simulink model "NHR9200Model4960_2020b_prog"  (R2020b)
settings: Solver=ode23tb  StartTime=0.0  StopTime=tFinal  FixedStep=Ts  MaxStep=0.2  RelTol=1e-3
values from neighbouring files (symbols this model uses):
  Imax_snk = 40    [nhr9200_runProg.m]
  Imax_snk_sfty = 80    [nhr9200_runProg.m]
  Imax_src = 10    [nhr9200_runProg.m]
  Imax_src_sfty = 25    [nhr9200_runProg.m]
  nhrLoad = 15    [nhr9200_runProg.m]
  op_state = 2    [nhr9200_runProg.m]
  Pmax_snk = 12    [nhr9200_runProg.m]
  Pmax_snk_sfty = 800    [nhr9200_runProg.m]
  Pmax_src = 8    [nhr9200_runProg.m]
  Pmax_src_sfty = 5000    [nhr9200_runProg.m]
  R_src = 0.001    [nhr9200_runProg.m]
  slew_i = 10    [nhr9200_runProg.m]
  slew_p = 300    [nhr9200_runProg.m]
  slew_r = 400    [nhr9200_runProg.m]
  slew_v = 200    [nhr9200_runProg.m]
  t_Imax_snk_sfty = 2    [nhr9200_runProg.m]
  t_Imax_src_sfty = 0.5    [nhr9200_runProg.m]
  t_Pmax_snk_sfty = 2    [nhr9200_runProg.m]
  t_Pmax_src_sfty = 2    [nhr9200_runProg.m]
  t_Vmax_gb = 2    [nhr9200_runProg.m]
  t_Vmin_gb = 2    [nhr9200_runProg.m]
  turn_on = 1    [nhr9200_runProg.m]
  v_bat = 0    [nhr9200_runProg.m]
  Vmax_gb = 800    [nhr9200_runProg.m]
  Vmax_src = 480    [nhr9200_runProg.m]
  Vmin_gb = -50    [nhr9200_runProg.m]
  Vmin_snk = 20    [nhr9200_runProg.m]
libraries: simulink x31, fl_lib x15, nesl_utility x14, simulink_extras x6, powerlib_meascontrol x6, ee_lib x2
(part 1 of 2)
settings Model: Creator=opal  LastModifiedBy=mne4
settings DataIOCC: ReturnWorkspaceOutputs=off
settings DebuggingCC: ParameterPrecisionLossMsg=none  UnconnectedInputMsg=none  UnconnectedOutputMsg=none  UnconnectedLineMsg=none  ArithmeticOperatorsInVariantConditions=warning
settings SFSimCC: SimUseLocalCustomCode=off  CustomCodeUndefinedFunction=UseInterfaceOnly
settings RTWCC: RTWUseLocalCustomCode=off
settings CodeAppCC: StateflowObjectComments=on
settings SimscapeCC: SimscapeNormalizeSystem=off

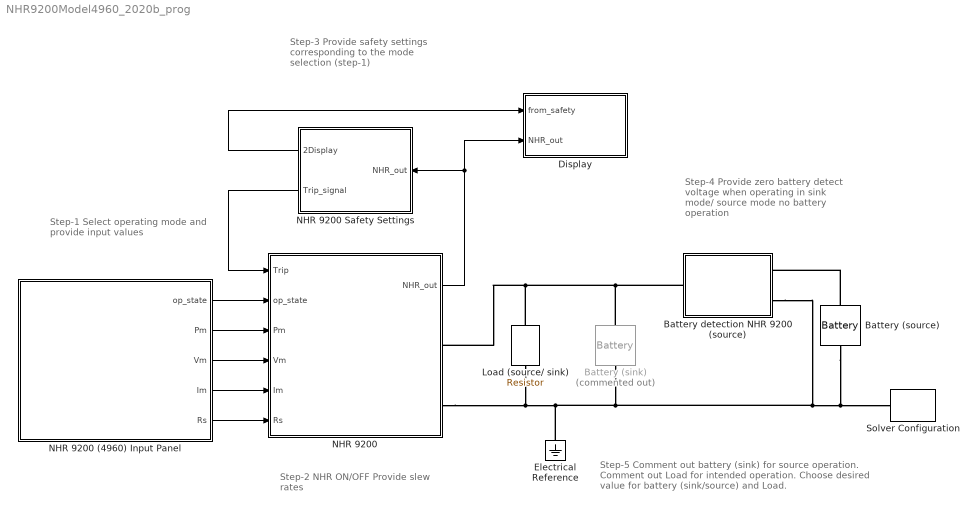
== system NHR9200Model4960_2020b_prog ==
  note: Step-1
      | Select operating mode and provide input values
  note: Step-2
      | NHR ON/OFF
      | Provide slew rates
  note: Step-3
      | Provide safety settings corresponding to the mode selection (step-1)
  note: Step-4
      | Provide zero battery detect voltage when operating in sink mode/ source mode no battery operation
  note: Step-5
      | Comment out battery (sink) for source operation.
      | Comment out Load for intended operation.
      | Choose desired value for battery (sink/source) and Load.
  Battery (sink) : ee_lib/Sources/Battery  Commented=on  Vnom=v_nom_bat_snk V  prm_dir=1  R1_dis=2 Ohm  R1_ch=2 Ohm  R1=r_bat_snk Ohm  prm_AH=1  AH=50 hr*A  V1=11.5 V  AH1=25 hr*A  prm_R2=1  R2=2000 Ohm  prm_dyn=1  Rp1=0.005 Ohm  tau1=30 s  Rp2=0.005 Ohm  tau2=30 s  Rp3=0.005 Ohm  tau3=30 s  Rp4=0.005 Ohm  tau4=30 s  Rp5=0.005 Ohm  tau5=30 s  prm_fade=1  N_fade=100  AH_fade=45 hr*A  R1_fade=2.02 Ohm  R1_ch_fade=2.02 Ohm  V1_fade=10.35 V  i_specify=off  i_priority=None  i=0 A  i_nominal_specify=off  i_nominal_unit=A  i_nominal_value=1  v_specify=off  v_priority=None  v=0 V  v_nominal_specify=off  v_nominal_unit=V  v_nominal_value=1  charge_specify=off  charge_priority=High  charge=50 hr*A  charge_nominal_specify=off  charge_nominal_unit=hr*A  charge_nominal_value=1  num_cycles_specify=off  num_cycles_priority=High  num_cycles=0  num_cycles_nominal_specify=off  num_cycles_nominal_unit=1  num_cycles_nominal_value=1  thermal_mass=30000 J/K  Tmeas=298.15 K  Vnom_T2=12 V  R1_T2=2.2 Ohm  R1_T2_dis=2.2 Ohm  R1_T2_ch=2.2 Ohm  V1_T2=11.4 V  R2_T2=2200 Ohm  Rp1_T2=0.005 Ohm  tau1_T2=30 s  Rp2_T2=0.005 Ohm  tau2_T2=30 s  Rp3_T2=0.005 Ohm  tau3_T2=30 s  Rp4_T2=0.005 Ohm  tau4_T2=30 s  Rp5_T2=0.005 Ohm  tau5_T2=30 s  Tmeas2=273.15 K  temperature_specify=off  temperature_priority=High  temperature=298.15 K  temperature_nominal_specify=off  temperature_nominal_unit=K  temperature_nominal_value=1
  Battery (source) : ee_lib/Sources/Battery  Vnom=v_nom_bat_src V  prm_dir=1  R1_dis=2 Ohm  R1_ch=2 Ohm  R1=r_bat_src Ohm  prm_AH=1  AH=50 hr*A  V1=11.5 V  AH1=25 hr*A  prm_R2=1  R2=2000 Ohm  prm_dyn=1  Rp1=0.005 Ohm  tau1=30 s  Rp2=0.005 Ohm  tau2=30 s  Rp3=0.005 Ohm  tau3=30 s  Rp4=0.005 Ohm  tau4=30 s  Rp5=0.005 Ohm  tau5=30 s  prm_fade=1  N_fade=100  AH_fade=45 hr*A  R1_fade=2.02 Ohm  R1_ch_fade=2.02 Ohm  V1_fade=10.35 V  i_specify=off  i_priority=None  i=0 A  i_nominal_specify=off  i_nominal_unit=A  i_nominal_value=1  v_specify=off  v_priority=None  v=0 V  v_nominal_specify=off  v_nominal_unit=V  v_nominal_value=1  charge_specify=off  charge_priority=High  charge=50 hr*A  charge_nominal_specify=off  charge_nominal_unit=hr*A  charge_nominal_value=1  num_cycles_specify=off  num_cycles_priority=High  num_cycles=0  num_cycles_nominal_specify=off  num_cycles_nominal_unit=1  num_cycles_nominal_value=1  thermal_mass=30000 J/K  Tmeas=298.15 K  Vnom_T2=12 V  R1_T2=2.2 Ohm  R1_T2_dis=2.2 Ohm  R1_T2_ch=2.2 Ohm  V1_T2=11.4 V  R2_T2=2200 Ohm  Rp1_T2=0.005 Ohm  tau1_T2=30 s  Rp2_T2=0.005 Ohm  tau2_T2=30 s  Rp3_T2=0.005 Ohm  tau3_T2=30 s  Rp4_T2=0.005 Ohm  tau4_T2=30 s  Rp5_T2=0.005 Ohm  tau5_T2=30 s  Tmeas2=273.15 K  temperature_specify=off  temperature_priority=High  temperature=298.15 K  temperature_nominal_specify=off  temperature_nominal_unit=K  temperature_nominal_value=1
  Battery detection NHR 9200 (source) : Subsystem  mask{Vdetect=v_bat}
      mask prompts: Vdetect "Battery detect voltage: (0: battery detection disabled)"
  Display : Subsystem
  Electrical Reference : fl_lib/Electrical/Electrical Elements/Electrical Reference
  Load (source/ sink) : fl_lib/Electrical/Electrical Elements/Resistor  R=nhrLoad Ohm  i_specify=off  i_priority=None  i=0 A  i_nominal_specify=off  i_nominal_unit=A  i_nominal_value=1  v_specify=off  v_priority=None  v=0 V  v_nominal_specify=off  v_nominal_unit=V  v_nominal_value=1
  NHR 9200 : Subsystem  mask{p_switch=turn_on, Vslew=slew_v, Islew=slew_i, Rslew=slew_r, Pslew=slew_p, Vbset=v_bat}
      mask prompts: p_switch "Enter 1 to turn ON, 0 to turn OFF NHR 9200"
      mask DialogControl DescTextVar Prompt: NHR 9200
      mask DialogControl Container5 Prompt: Slew Rates
      mask DialogControl control2 Prompt: Voltage slew rate [0.165V/s-600V/ms]:
      mask DialogControl Control3 Prompt: Current slew rate [0.011 A/s-40A/ms]:
      mask DialogControl Control4 Prompt: Resistance slew rate [0.14 ohms/s-500 ohms/ms]:
      mask DialogControl Control5 Prompt: Power slew rate [2W/s-8kW/s]:
      mask DialogControl Container6 Prompt: Set Battery Detect Voltage
      mask DialogControl Control7 Prompt: Battery detect voltage: (0: battery detection disabled)
      mask Display: image('NHR9200.png');
  NHR 9200 (4960) Input Panel : Subsystem  mask{op_state=op_state, Vmch=Vmax_src, Imch=Imax_src, Pmch=Pmax_src, Rsch=R_src, Vmdch=Vmin_snk, Imdch=Imax_snk, Pmdch=Pmax_snk}
      mask DialogControl Control2 Prompt: Select operating state (1: standby, 2: Charge, 3: Discharge, 4: Battery)
      mask DialogControl Container7 Prompt: Limiting mode (CV, CC, CP, CR)
      mask DialogControl Container9 Prompt: Set '0' to disable a mode
      mask DialogControl Container4 Prompt: Charging mode input parameters
      mask DialogControl Control3 Prompt: Max Voltage [0~600V]:
      mask DialogControl Control4 Prompt: Max Current [0~(+40)A]:
      mask DialogControl Control5 Prompt: Max Power [0~8kW]:
      mask DialogControl Control6 Prompt: Resistance [0~500 ohms]:
      mask DialogControl Container4_copy Prompt: Discharging mode input parameters
      mask DialogControl Control3_copy Prompt: Min Voltage [10~600V]:
      mask DialogControl Control4_copy Prompt: Max Current [0~(-40)A], enter absolute value:
      mask DialogControl Control5_copy Prompt: Max Power [0~12kW]:
      mask Display: image('NHR9200Model4960HMI.png');
  NHR 9200 Safety Settings : Subsystem  mask{Vmin=Vmin_gb, Tvmin=t_Vmin_gb, Vmax=Vmax_gb, Tvmax=t_Vmax_gb, Imaxdch=Imax_snk_sfty, Timaxdch=t_Imax_snk_sfty, Pmaxdch=Pmax_snk_sfty, Tpmaxdch=t_Pmax_snk_sfty, Imaxch=Imax_src_sfty, Timaxch=t_Imax_src_sfty, Pmaxch=Pmax_src_sfty, Tpmaxch=t_Pmax_src_sfty}
      mask prompts: Vmin "Min Voltage (V):"; Tvmin "Min Voltage time (S):"; Vmax "Max Voltage (V):"; Tvmax "Max Voltage time (S):"; Imaxdch "Max Current (A):"; Timaxdch "Max Current Time (S):"; Pmaxdch "Max Power (W):"; Tpmaxdch "Max Power Time (S):"; Imaxch "Max Current (A):"; Timaxch "Max Current Time (S):"; Pmaxch "Max Power (W):"; Tpmaxch "Max Power Time (S):"
      mask DialogControl DescTextVar Prompt: NHR 9410 Safety Settings
      mask DialogControl Container27 Prompt: Provide safety trip parameters
      mask DialogControl Container123 Prompt: Global safety limits (all modes)
      mask DialogControl Container124 Prompt: Discharge safety limits (sink mode- discharge and battery)
      mask DialogControl Container125 Prompt: Charge safety limits (source mode- charge and battery)
  Solver Configuration : nesl_utility/Solver Configuration  PhysicalDomain=network_engine_domain  SubClassName=solver  LeftPortType=input  RightPortType=generic  Tones=[]  Harmonics=[]  SimulateNoise=off  Profile=off  UseLocalSampling=off  EnableSwitchedLinearOptims=on  FrequencyDomain=off  UseCCode=off  RelTol=0.001  AbsTol=1e-06  MinStep=1e-09  ToWorkspace=off  RevertToSquareIcSolve=off  NumHomotopyIterations=100  PhasorMode=off  PhasorModeNumHarmonics=1  DoDC=off  ResidualTolerance=1e-09  UseLocalSolver=on  LocalSolverChoice=NE_TRAPEZOIDAL_ADVANCER  LocalSolverSampleTime=Ts  DoFixedCost=off  MaxNonlinIter=3  MaxModeIter=2  ComputeImpulses=off  ImpulseIterations=2  LinearAlgebra=Sparse  EquationFormulation=NE_TIME_EF  DelaysMemoryBudget=1024  AutomaticFiltering=off  FilteringTimeConstant=0.001  PartitionStorageMethod=AS_NEEDED  PartitionMemoryBudget=1024  PartitionMethod=FAST
  wires:
  NHR 9200/1(NHR_out) -> Display/2(NHR_out), NHR 9200 Safety Settings/1(NHR_out)
  NHR 9200 Safety Settings/2(Trip_signal) -> NHR 9200/1(Trip)
  NHR 9200 (4960) Input Panel/1(op_state) -> NHR 9200/2(op_state)
  NHR 9200 (4960) Input Panel/2(Pm) -> NHR 9200/3(Pm)
  NHR 9200 (4960) Input Panel/3(Vm) -> NHR 9200/4(Vm)
  NHR 9200 (4960) Input Panel/4(Im) -> NHR 9200/5(Im)
  NHR 9200 (4960) Input Panel/5(Rs) -> NHR 9200/6(Rs)
  NHR 9200 Safety Settings/1(2Display) -> Display/1(from_safety)
  connections:
  Electrical Reference/LConn1 -- NHR 9200/RConn2 -- Load (source/ sink)/RConn1 -- Battery detection NHR 9200 (source)/LConn2 -- Battery (source)/RConn1 -- Solver Configuration/RConn1 -- Battery (sink)/RConn1
  Load (source/ sink)/LConn1 -- Battery (sink)/LConn1 -- Battery detection NHR 9200 (source)/RConn1 -- NHR 9200/RConn1
  Battery (source)/LConn1 -- Battery detection NHR 9200 (source)/LConn1

== system NHR9200Model4960_2020b_prog/Battery detection NHR 9200 (source) ==
  Battery detection : Subsystem
  Switch : fl_lib/Electrical/Electrical Elements/Switch  R_closed=1e-6 Ohm  G_open=1e-50 1/Ohm  Threshold=0.5  i_specify=off  i_priority=None  i=0 A  i_nominal_specify=off  i_nominal_unit=A  i_nominal_value=1  v_specify=off  v_priority=None  v=0 V  v_nominal_specify=off  v_nominal_unit=V  v_nominal_value=1
  Voltage Sensor : fl_lib/Electrical/Electrical Sensors/Voltage Sensor
  +in : PMIOPort  Side=Right
  +out2battery : PMIOPort  Port=2  Side=Left
  - : PMIOPort  Port=3  Side=Left
  connections:
  Voltage Sensor/LConn1 -- +out2battery/RConn1 -- Switch/LConn1
  Battery detection/LConn1 -- Voltage Sensor/RConn1
  Switch/RConn2 -- +in/RConn1
  Battery detection/RConn1 -- Switch/RConn1
  Voltage Sensor/RConn2 -- -/RConn1

== system NHR9200Model4960_2020b_prog/Display ==
  note: Pmax_trip (charge)
  note: Imax_trip (charge)
  note: Pmax_trip (discharge)
  note: Imax_trip (discharge)
  note: Vmax_trip
  note: Vmin_trip
  note: Trip
  from_safety : Inport
  NHR_out : Inport  Port=2
  Demux : Demux
  Demux1 : Demux  Outputs=7
  Divide : Product  Commented=on  Inputs=*/
  Mux : Mux  Inputs=2
  NHR 9200 output waveforms [P,V,I] : Scope  NumInputPorts=3
  R : Scope  Commented=on
  Terminator : Terminator
  Trip Signals : Scope  NumInputPorts=7
  Vout/Vuut : Scope  NumInputPorts=2
  wires:
  Demux/1 -> NHR 9200 output waveforms [P,V,I]/1
  NHR_out/1 -> Demux/1
  from_safety/1 -> Demux1/1
  Demux1/1 -> Trip Signals/1
  Demux1/2 -> Trip Signals/2
  Demux1/3 -> Trip Signals/3
  Demux1/4 -> Trip Signals/4
  Demux1/5 -> Trip Signals/5
  Demux1/6 -> Trip Signals/6
  Demux1/7 -> Trip Signals/7
  Demux/4 -> Terminator/1
  Demux/2 -> Mux/1, Divide/1, NHR 9200 output waveforms [P,V,I]/2
  Divide/1 -> R/1
  Demux/3 -> Divide/2, NHR 9200 output waveforms [P,V,I]/3
  [Vuut_bat] -> Mux/2
  [Vdetect] -> Vout/Vuut/2
  Mux/1 -> Vout/Vuut/1

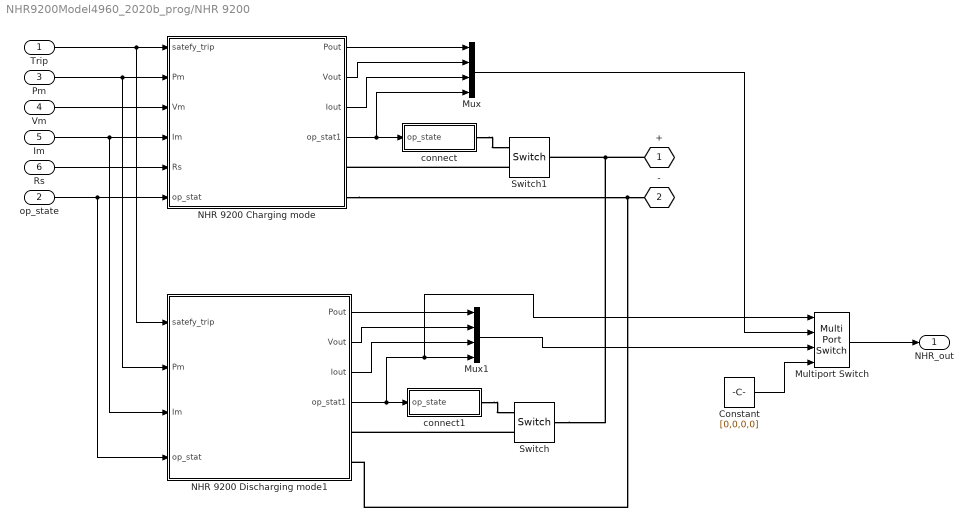
== system NHR9200Model4960_2020b_prog/NHR 9200 ==
  Trip : Inport
  op_state : Inport  Port=2
  Pm : Inport  Port=3
  Vm : Inport  Port=4
  Im : Inport  Port=5
  Rs : Inport  Port=6
  Constant : Constant  Value=[0,0,0,0]
  Multiport Switch : MultiPortSwitch  DataPortOrder=Specify indices  Inputs=2  DataPortIndices={2,3}  DataPortForDefault=Additional data port  DiagnosticForDefault=None
  Mux : Mux
  Mux1 : Mux
  NHR 9200 Charging mode : Subsystem
  NHR 9200 Discharging mode1 : Subsystem
  Switch : fl_lib/Electrical/Electrical Elements/Switch  R_closed=1e-6 Ohm  G_open=1e-50 1/Ohm  Threshold=0.5  i_specify=off  i_priority=None  i=0 A  i_nominal_specify=off  i_nominal_unit=A  i_nominal_value=1  v_specify=off  v_priority=None  v=0 V  v_nominal_specify=off  v_nominal_unit=V  v_nominal_value=1
  Switch1 : fl_lib/Electrical/Electrical Elements/Switch  R_closed=1e-6 Ohm  G_open=1e-50 1/Ohm  Threshold=0.5  i_specify=off  i_priority=None  i=0 A  i_nominal_specify=off  i_nominal_unit=A  i_nominal_value=1  v_specify=off  v_priority=None  v=0 V  v_nominal_specify=off  v_nominal_unit=V  v_nominal_value=1
  connect : Subsystem  mask{op_state=2}
      mask prompts: op_state "Intended operating state (integer number):"
      mask DialogControl Control3 Prompt: Select operating state (1: standby, 2: Charge, 3: Discharge, 4: Battery)
  connect1 : Subsystem  mask{op_state=3}
      mask prompts: op_state "Intended operating state (integer number):"
      mask DialogControl Control3 Prompt: Select operating state (1: standby, 2: Charge, 3: Discharge, 4: Battery)
  + : PMIOPort  Side=Right
  - : PMIOPort  Port=2  Side=Right
  NHR_out : Outport  VectorParamsAs1DForOutWhenUnconnected=off
  wires:
  Vm/1 -> NHR 9200 Charging mode/3(Vm)
  Im/1 -> NHR 9200 Discharging mode1/3(Im), NHR 9200 Charging mode/4(Im)
  Rs/1 -> NHR 9200 Charging mode/5(Rs)
  NHR 9200 Charging mode/1(Pout) -> Mux/1
  NHR 9200 Charging mode/2(Vout) -> Mux/2
  NHR 9200 Charging mode/3(Iout) -> Mux/3
  op_state/1 -> NHR 9200 Discharging mode1/4("op_stat "), NHR 9200 Charging mode/6("op_stat ")
  Trip/1 -> NHR 9200 Discharging mode1/1(satefy_trip), NHR 9200 Charging mode/1(satefy_trip)
  NHR 9200 Charging mode/4(op_stat1) -> Mux/4, connect/1(op_state)
  Pm/1 -> NHR 9200 Discharging mode1/2(Pm), NHR 9200 Charging mode/2(Pm)
  NHR 9200 Discharging mode1/4(op_stat1) -> Mux1/4, Multiport Switch/1, connect1/1(op_state)
  NHR 9200 Discharging mode1/3(Iout) -> Mux1/3
  NHR 9200 Discharging mode1/2(Vout) -> Mux1/2
  NHR 9200 Discharging mode1/1(Pout) -> Mux1/1
  Multiport Switch/1 -> NHR_out/1
  Mux1/1 -> Multiport Switch/3
  Mux/1 -> Multiport Switch/2
  Constant/1 -> Multiport Switch/4
  connections:
  NHR 9200 Discharging mode1/RConn2 -- NHR 9200 Charging mode/RConn2 -- -/RConn1
  +/RConn1 -- Switch/LConn1 -- Switch1/LConn1
  Switch1/RConn2 -- NHR 9200 Charging mode/RConn1
  connect/RConn1 -- Switch1/RConn1
  connect1/RConn1 -- Switch/RConn1
  Switch/RConn2 -- NHR 9200 Discharging mode1/RConn1

== system NHR9200Model4960_2020b_prog/NHR 9200 (4960) Input Panel ==
  Charging mode Input Params : Subsystem
  Compare To Constant1 : simulink/Logic and Bit Operations/Compare To Constant  relop===  const=3  OutDataTypeStr=boolean
  Compare To Constant4 : simulink/Logic and Bit Operations/Compare To Constant  relop===  const=2  OutDataTypeStr=boolean
  Constant : Constant  Value=op_state
  Constant1 : Constant  Value=[0,0,0,0]
  Demux : Demux
  Discharging mode Input Params : Subsystem
  Multiport Switch : MultiPortSwitch  DataPortOrder=Specify indices  Inputs=2  DataPortIndices={2,3}  DataPortForDefault=Additional data port  DiagnosticForDefault=None
  Mux : Mux
  Mux1 : Mux
  op_state : Outport  VectorParamsAs1DForOutWhenUnconnected=off
  Pm : Outport  Port=2  VectorParamsAs1DForOutWhenUnconnected=off
  Vm : Outport  Port=3  VectorParamsAs1DForOutWhenUnconnected=off
  Im : Outport  Port=4  VectorParamsAs1DForOutWhenUnconnected=off
  Rs : Outport  Port=5  VectorParamsAs1DForOutWhenUnconnected=off
  wires:
  Compare To Constant4/1 -> Charging mode Input Params/Enable
  Constant/1 -> Compare To Constant1/1, Multiport Switch/1, op_state/1, Compare To Constant4/1
  Demux/1 -> Vm/1
  Demux/2 -> Im/1
  Demux/3 -> Pm/1
  Demux/4 -> Rs/1
  Multiport Switch/1 -> Demux/1
  Charging mode Input Params/1(Vm) -> Mux/1
  Charging mode Input Params/2(Im) -> Mux/2
  Charging mode Input Params/3(Pm) -> Mux/3
  Charging mode Input Params/4(Rs) -> Mux/4
  Mux/1 -> Multiport Switch/2
  Discharging mode Input Params/1(Vm) -> Mux1/1
  Discharging mode Input Params/2(Im) -> Mux1/2
  Discharging mode Input Params/3(Pm) -> Mux1/3
  Discharging mode Input Params/4(Rs) -> Mux1/4
  Mux1/1 -> Multiport Switch/3
  Constant1/1 -> Multiport Switch/4
  Compare To Constant1/1 -> Discharging mode Input Params/Enable

== system NHR9200Model4960_2020b_prog/NHR 9200 Safety Settings ==
  NHR_out : Inport
  Charge safety limits : Subsystem
      settings: MinAlgLoopOccurrences=on
  Compare To Constant1 : simulink/Logic and Bit Operations/Compare To Constant  relop===  const=4  OutDataTypeStr=boolean
  Compare To Constant2 : simulink/Logic and Bit Operations/Compare To Constant  relop===  const=3  OutDataTypeStr=boolean
  Compare To Constant3 : simulink/Logic and Bit Operations/Compare To Constant  relop===  const=4  OutDataTypeStr=boolean
  Compare To Constant4 : simulink/Logic and Bit Operations/Compare To Constant  relop===  const=2  OutDataTypeStr=boolean
  Data Type Conversion : DataTypeConversion  OutDataTypeStr=double
  Demux : Demux
  Discharge safety limits : Subsystem
      settings: MinAlgLoopOccurrences=on
  Global safety limits : Subsystem
  Logical Operator1 : Logic  Operator=OR  AllPortsSameDT=off  OutDataTypeStr=boolean
  Logical Operator2 : Logic  Operator=OR  AllPortsSameDT=off  OutDataTypeStr=boolean
  Logical Operator3 : Logic  Operator=OR  Inputs=6  AllPortsSameDT=off  OutDataTypeStr=boolean
  Mux : Mux  Inputs=7
  Unit Delay2 : UnitDelay  InitialCondition=1  SampleTime=-1  HasFrameUpgradeWarning=on
  2Display : Outport  VectorParamsAs1DForOutWhenUnconnected=off
  Trip_signal : Outport  Port=2  VectorParamsAs1DForOutWhenUnconnected=off
  wires:
  NHR_out/1 -> Demux/1
  Logical Operator3/1 -> Mux/1, Data Type Conversion/1
  Compare To Constant2/1 -> Logical Operator1/1
  Compare To Constant1/1 -> Logical Operator1/2
  Logical Operator1/1 -> Discharge safety limits/Enable
  Compare To Constant3/1 -> Logical Operator2/2
  Compare To Constant4/1 -> Logical Operator2/1
  Logical Operator2/1 -> Charge safety limits/Enable
  Demux/4 -> Compare To Constant2/1, Compare To Constant1/1, Compare To Constant3/1, Compare To Constant4/1
  Global safety limits/1(Vmin_trip) -> Mux/2, Logical Operator3/1
  Global safety limits/2(Vmax_trip1) -> Mux/3, Logical Operator3/2
  Discharge safety limits/1(I_trip) -> Mux/4, Logical Operator3/3
  Discharge safety limits/2(P_trip) -> Mux/5, Logical Operator3/4
  Charge safety limits/1(I_trip) -> Mux/6, Logical Operator3/5
  Charge safety limits/2(P_trip) -> Mux/7, Logical Operator3/6
  Demux/1 -> Charge safety limits/2(P), Discharge safety limits/2(P)
  Demux/2 -> Global safety limits/1(V)
  Demux/3 -> Charge safety limits/1(I), Discharge safety limits/1(I)
  Mux/1 -> 2Display/1
  Data Type Conversion/1 -> Unit Delay2/1
  Unit Delay2/1 -> Trip_signal/1

== system NHR9200Model4960_2020b_prog/Battery detection NHR 9200 (source)/Battery detection ==
  Compare To Constant : simulink/Logic and Bit Operations/Compare To Constant  relop=>=  const=Vdetect  OutDataTypeStr=uint8
  Compare To Constant1 : simulink/Logic and Bit Operations/Compare To Constant  relop===  const=0  OutDataTypeStr=boolean
  Constant : Constant  Value=Vdetect
  Constant1 : Constant  Value=0
  Data Type Conversion : DataTypeConversion  OutDataTypeStr=double
  PS-Simulink Converter3 : nesl_utility/PS-Simulink Converter  PhysicalDomain=network_engine_domain  SubClassName=ps_output  LeftPortType=input  RightPortType=output  PseudoPeriodic=off  Frequencies=[]  Unit=1  AffineConversion=off
  Simulink-PS Converter : nesl_utility/Simulink-PS Converter  PhysicalDomain=network_engine_domain  SubClassName=ps_input  LeftPortType=input  RightPortType=output  PseudoPeriodic=off  Frequencies=[]  NoiseDistribution=none  NoiseParameters=[]  Unit=1  AffineConversion=off  FilteringAndDerivatives=provide  SimscapeFilterOrder=1  InputFilterTimeConstant=0.001  UdotUserProvided=0
  Switch : Switch  Criteria=u2 > Threshold
  Unit Delay2 : UnitDelay  InitialCondition=1  SampleTime=-1  HasFrameUpgradeWarning=on
  2Switch : PMIOPort  Side=Right
  V : PMIOPort  Port=2  Side=Left
  tag scope: Vdetect=global, Vuut_bat=global
  wires:
  Compare To Constant1/1 -> Switch/2
  Switch/1 -> Data Type Conversion/1, [Vdetect]
  Constant/1 -> Compare To Constant1/1
  Constant1/1 -> Switch/1
  Compare To Constant/1 -> Unit Delay2/1
  Data Type Conversion/1 -> Simulink-PS Converter/1
  PS-Simulink Converter3/1 -> Compare To Constant/1, [Vuut_bat]
  Unit Delay2/1 -> Switch/3
  connections:
  Simulink-PS Converter/RConn1 -- 2Switch/RConn1
  PS-Simulink Converter3/LConn1 -- V/RConn1

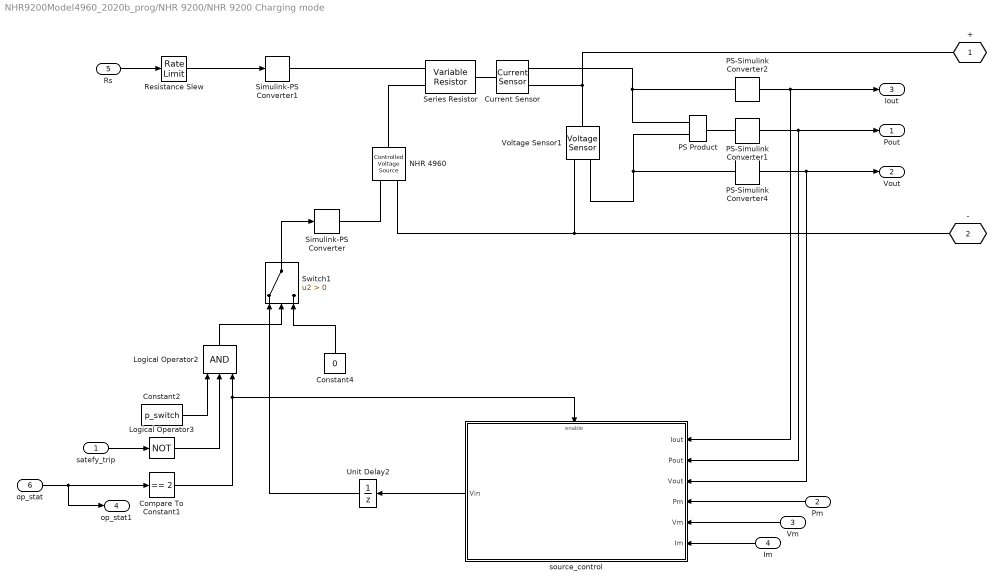
== system NHR9200Model4960_2020b_prog/NHR 9200/NHR 9200 Charging mode ==
  satefy_trip : Inport
  Pm : Inport  Port=2
  Vm : Inport  Port=3
  Im : Inport  Port=4
  Rs : Inport  Port=5
  "op_stat " : Inport  Port=6
  Compare To Constant1 : simulink/Logic and Bit Operations/Compare To Constant  relop===  const=2  OutDataTypeStr=boolean
  Constant2 : Constant  Value=p_switch
  Constant4 : Constant  Value=0
  Current Sensor : fl_lib/Electrical/Electrical Sensors/Current Sensor
  Logical Operator2 : Logic  Inputs=3  AllPortsSameDT=off  OutDataTypeStr=boolean
  Logical Operator3 : Logic  Operator=NOT  AllPortsSameDT=off  OutDataTypeStr=boolean
  NHR 4960 : fl_lib/Electrical/Electrical Sources/Controlled Voltage Source
  PS Product : fl_lib/Physical Signals/Functions/PS Product
  PS-Simulink Converter1 : nesl_utility/PS-Simulink Converter  PhysicalDomain=network_engine_domain  SubClassName=ps_output  LeftPortType=input  RightPortType=output  PseudoPeriodic=off  Frequencies=[]  Unit=inherit  AffineConversion=off
  PS-Simulink Converter2 : nesl_utility/PS-Simulink Converter  PhysicalDomain=network_engine_domain  SubClassName=ps_output  LeftPortType=input  RightPortType=output  PseudoPeriodic=off  Frequencies=[]  Unit=1  AffineConversion=off
  PS-Simulink Converter4 : nesl_utility/PS-Simulink Converter  PhysicalDomain=network_engine_domain  SubClassName=ps_output  LeftPortType=input  RightPortType=output  PseudoPeriodic=off  Frequencies=[]  Unit=1  AffineConversion=off
  Resistance Slew : RateLimiter  RisingSlewLimit=Rslew  FallingSlewLimit=-Rslew
  Series Resistor : fl_lib/Electrical/Electrical Elements/Variable Resistor  Rmin=0 Ohm  i_specify=off  i_priority=None  i=0 A  i_nominal_specify=off  i_nominal_unit=A  i_nominal_value=1  v_specify=off  v_priority=None  v=0 V  v_nominal_specify=off  v_nominal_unit=V  v_nominal_value=1
  Simulink-PS Converter : nesl_utility/Simulink-PS Converter  PhysicalDomain=network_engine_domain  SubClassName=ps_input  LeftPortType=input  RightPortType=output  PseudoPeriodic=off  Frequencies=[]  NoiseDistribution=none  NoiseParameters=[]  Unit=1  AffineConversion=off  FilteringAndDerivatives=filter  SimscapeFilterOrder=1  InputFilterTimeConstant=0.001  UdotUserProvided=0
  Simulink-PS Converter1 : nesl_utility/Simulink-PS Converter  PhysicalDomain=network_engine_domain  SubClassName=ps_input  LeftPortType=input  RightPortType=output  PseudoPeriodic=off  Frequencies=[]  NoiseDistribution=none  NoiseParameters=[]  Unit=1  AffineConversion=off  FilteringAndDerivatives=filter  SimscapeFilterOrder=1  InputFilterTimeConstant=0.001  UdotUserProvided=0
  Switch1 : Switch  Criteria=u2 > Threshold  SaturateOnIntegerOverflow=on
  Unit Delay2 : UnitDelay  InitialCondition=1  SampleTime=-1  HasFrameUpgradeWarning=on
  Voltage Sensor1 : fl_lib/Electrical/Electrical Sensors/Voltage Sensor
  source_control : Subsystem
  + : PMIOPort  Tag=PMCPort  Side=Right
  - : PMIOPort  Tag=PMCPort  Port=2  Side=Right
  Pout : Outport  VectorParamsAs1DForOutWhenUnconnected=off
  Vout : Outport  Port=2  VectorParamsAs1DForOutWhenUnconnected=off
  Iout : Outport  Port=3  VectorParamsAs1DForOutWhenUnconnected=off
  op_stat1 : Outport  Port=4  VectorParamsAs1DForOutWhenUnconnected=off
  wires:
  PS-Simulink Converter2/1 -> Iout/1, source_control/1(Iout)
  PS-Simulink Converter1/1 -> Pout/1, source_control/2(Pout)
  PS-Simulink Converter4/1 -> Vout/1, source_control/3(Vout)
  Rs/1 -> Resistance Slew/1
  Resistance Slew/1 -> Simulink-PS Converter1/1
  Pm/1 -> source_control/4(Pm)
  Vm/1 -> source_control/5(Vm)
  Im/1 -> source_control/6(Im)
  satefy_trip/1 -> Logical Operator3/1
  "op_stat "/1 -> op_stat1/1, Compare To Constant1/1
  Constant4/1 -> Switch1/3
  Logical Operator3/1 -> Logical Operator2/2
  Logical Operator2/1 -> Switch1/2
  Compare To Constant1/1 -> Logical Operator2/3, source_control/Enable
  source_control/1(Vin) -> Unit Delay2/1
  Constant2/1 -> Logical Operator2/1
  Switch1/1 -> Simulink-PS Converter/1
  Unit Delay2/1 -> Switch1/1
  connections:
  Simulink-PS Converter1/RConn1 -- Series Resistor/LConn1
  Series Resistor/LConn2 -- NHR 4960/LConn1
  Current Sensor/LConn1 -- Series Resistor/RConn1
  -/RConn1 -- NHR 4960/RConn2 -- Voltage Sensor1/RConn2
  PS-Simulink Converter2/LConn1 -- PS Product/LConn1 -- Current Sensor/RConn1
  Voltage Sensor1/LConn1 -- +/RConn1 -- Current Sensor/RConn2
  PS Product/RConn1 -- PS-Simulink Converter1/LConn1
  Voltage Sensor1/RConn1 -- PS Product/LConn2 -- PS-Simulink Converter4/LConn1
  Simulink-PS Converter/RConn1 -- NHR 4960/RConn1

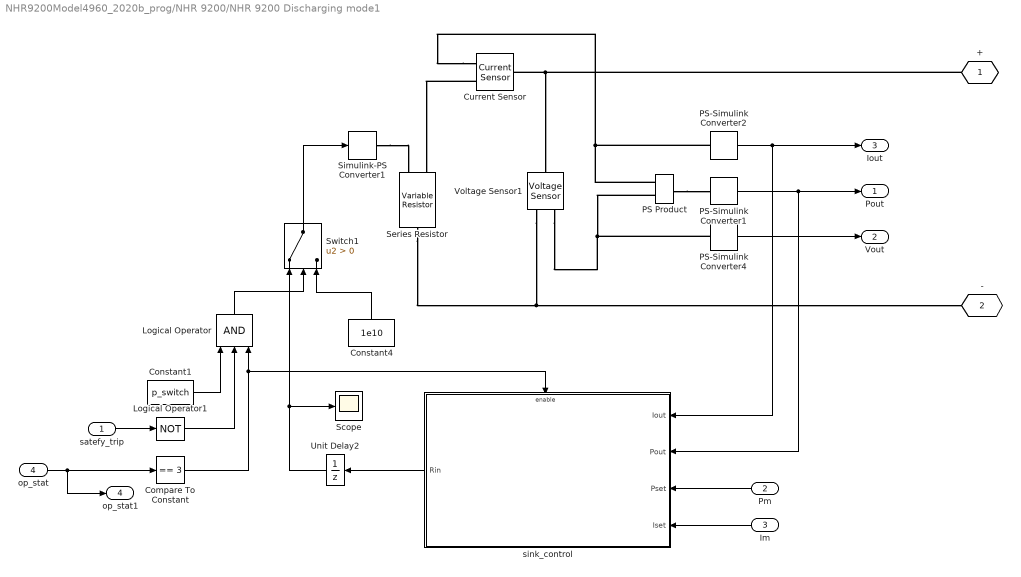
== system NHR9200Model4960_2020b_prog/NHR 9200/NHR 9200 Discharging mode1 ==
  satefy_trip : Inport
  Pm : Inport  Port=2
  Im : Inport  Port=3
  "op_stat " : Inport  Port=4
  Compare To Constant : simulink/Logic and Bit Operations/Compare To Constant  relop===  const=3  OutDataTypeStr=boolean
  Constant1 : Constant  Value=p_switch
  Constant4 : Constant  Value=1e10
  Current Sensor : fl_lib/Electrical/Electrical Sensors/Current Sensor
  Logical Operator : Logic  Inputs=3  AllPortsSameDT=off  OutDataTypeStr=boolean
  Logical Operator1 : Logic  Operator=NOT  AllPortsSameDT=off  OutDataTypeStr=boolean
  PS Product : fl_lib/Physical Signals/Functions/PS Product
  PS-Simulink Converter1 : nesl_utility/PS-Simulink Converter  PhysicalDomain=network_engine_domain  SubClassName=ps_output  LeftPortType=input  RightPortType=output  PseudoPeriodic=off  Frequencies=[]  Unit=inherit  AffineConversion=off
  PS-Simulink Converter2 : nesl_utility/PS-Simulink Converter  PhysicalDomain=network_engine_domain  SubClassName=ps_output  LeftPortType=input  RightPortType=output  PseudoPeriodic=off  Frequencies=[]  Unit=1  AffineConversion=off
  PS-Simulink Converter4 : nesl_utility/PS-Simulink Converter  PhysicalDomain=network_engine_domain  SubClassName=ps_output  LeftPortType=input  RightPortType=output  PseudoPeriodic=off  Frequencies=[]  Unit=1  AffineConversion=off
  Scope : Scope
  Series Resistor : fl_lib/Electrical/Electrical Elements/Variable Resistor  Rmin=1e-3 Ohm  i_specify=off  i_priority=None  i=0 A  i_nominal_specify=off  i_nominal_unit=A  i_nominal_value=1  v_specify=off  v_priority=None  v=0 V  v_nominal_specify=off  v_nominal_unit=V  v_nominal_value=1
  Simulink-PS Converter1 : nesl_utility/Simulink-PS Converter  PhysicalDomain=network_engine_domain  SubClassName=ps_input  LeftPortType=input  RightPortType=output  PseudoPeriodic=off  Frequencies=[]  NoiseDistribution=none  NoiseParameters=[]  Unit=1  AffineConversion=off  FilteringAndDerivatives=filter  SimscapeFilterOrder=1  InputFilterTimeConstant=0.001  UdotUserProvided=0
  Switch1 : Switch  Criteria=u2 > Threshold  SaturateOnIntegerOverflow=on
  Unit Delay2 : UnitDelay  InitialCondition=1  SampleTime=-1  HasFrameUpgradeWarning=on
  Voltage Sensor1 : fl_lib/Electrical/Electrical Sensors/Voltage Sensor
  sink_control : Subsystem
      settings: MinAlgLoopOccurrences=on
  + : PMIOPort  Tag=PMCPort  Side=Right
  - : PMIOPort  Tag=PMCPort  Port=2  Side=Right
  Pout : Outport  VectorParamsAs1DForOutWhenUnconnected=off
  Vout : Outport  Port=2  VectorParamsAs1DForOutWhenUnconnected=off
  Iout : Outport  Port=3  VectorParamsAs1DForOutWhenUnconnected=off
  op_stat1 : Outport  Port=4  VectorParamsAs1DForOutWhenUnconnected=off
  wires:
  "op_stat "/1 -> Compare To Constant/1, op_stat1/1
  Im/1 -> sink_control/4(Iset)
  Pm/1 -> sink_control/3(Pset)
  Constant1/1 -> Logical Operator/1
  satefy_trip/1 -> Logical Operator1/1
  Logical Operator1/1 -> Logical Operator/2
  PS-Simulink Converter4/1 -> Vout/1
  PS-Simulink Converter2/1 -> Iout/1, sink_control/1(Iout)
  Switch1/1 -> Simulink-PS Converter1/1
  Constant4/1 -> Switch1/3
  Logical Operator/1 -> Switch1/2
  Compare To Constant/1 -> sink_control/Enable, Logical Operator/3
  PS-Simulink Converter1/1 -> Pout/1, sink_control/2(Pout)
  sink_control/1(Rin) -> Unit Delay2/1
  Unit Delay2/1 -> Scope/1, Switch1/1
  connections:
  PS-Simulink Converter4/LConn1 -- PS Product/LConn2 -- Voltage Sensor1/RConn1
  PS Product/RConn1 -- PS-Simulink Converter1/LConn1
  +/RConn1 -- Voltage Sensor1/LConn1 -- Current Sensor/LConn1
  Current Sensor/RConn1 -- PS Product/LConn1 -- PS-Simulink Converter2/LConn1
  Voltage Sensor1/RConn2 -- -/RConn1 -- Series Resistor/RConn1
  Simulink-PS Converter1/RConn1 -- Series Resistor/LConn1
  Current Sensor/RConn2 -- Series Resistor/LConn2

== system NHR9200Model4960_2020b_prog/NHR 9200/connect ==
  op_state : Inport
  Compare To Constant2 : simulink/Logic and Bit Operations/Compare To Constant  relop===  const=op_state  OutDataTypeStr=boolean
  Data Type Conversion : DataTypeConversion  OutDataTypeStr=double
  Simulink-PS Converter : nesl_utility/Simulink-PS Converter  PhysicalDomain=network_engine_domain  SubClassName=ps_input  LeftPortType=input  RightPortType=output  PseudoPeriodic=off  Frequencies=[]  NoiseDistribution=none  NoiseParameters=[]  Unit=1  AffineConversion=off  FilteringAndDerivatives=provide  SimscapeFilterOrder=1  InputFilterTimeConstant=0.001  UdotUserProvided=0
  sw_on : PMIOPort  Side=Right
  wires:
  Compare To Constant2/1 -> Data Type Conversion/1
  Data Type Conversion/1 -> Simulink-PS Converter/1
  op_state/1 -> Compare To Constant2/1
  connections:
  Simulink-PS Converter/RConn1 -- sw_on/RConn1

== system NHR9200Model4960_2020b_prog/NHR 9200/connect1 ==
  op_state : Inport
  Compare To Constant2 : simulink/Logic and Bit Operations/Compare To Constant  relop===  const=op_state  OutDataTypeStr=boolean
  Data Type Conversion : DataTypeConversion  OutDataTypeStr=double
  Simulink-PS Converter : nesl_utility/Simulink-PS Converter  PhysicalDomain=network_engine_domain  SubClassName=ps_input  LeftPortType=input  RightPortType=output  PseudoPeriodic=off  Frequencies=[]  NoiseDistribution=none  NoiseParameters=[]  Unit=1  AffineConversion=off  FilteringAndDerivatives=provide  SimscapeFilterOrder=1  InputFilterTimeConstant=0.001  UdotUserProvided=0
  sw_on : PMIOPort  Side=Right
  wires:
  op_state/1 -> Compare To Constant2/1
  Data Type Conversion/1 -> Simulink-PS Converter/1
  Compare To Constant2/1 -> Data Type Conversion/1
  connections:
  Simulink-PS Converter/RConn1 -- sw_on/RConn1

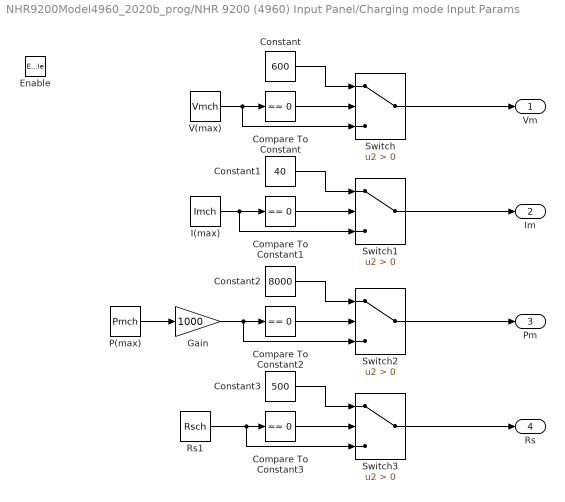
== system NHR9200Model4960_2020b_prog/NHR 9200 (4960) Input Panel/Charging mode Input Params ==
  Enable : EnablePort
  Compare To Constant{,1..3} (4 alike) : simulink/Logic and Bit Operations/Compare To Constant  relop===  const=0  OutDataTypeStr=boolean
  Constant : Constant  Value=600
  Constant1 : Constant  Value=40
  Constant2 : Constant  Value=8000
  Constant3 : Constant  Value=500
  Gain : Gain  Gain=1000
  I(max) : Constant  Value=Imch
  P(max) : Constant  Value=Pmch
  Rs1 : Constant  Value=Rsch
  Switch{,1..3} (4 alike) : Switch  Criteria=u2 > Threshold
  V(max) : Constant  Value=Vmch
  Vm : Outport  VectorParamsAs1DForOutWhenUnconnected=off
  Im : Outport  Port=2  VectorParamsAs1DForOutWhenUnconnected=off
  Pm : Outport  Port=3  VectorParamsAs1DForOutWhenUnconnected=off
  Rs : Outport  Port=4  VectorParamsAs1DForOutWhenUnconnected=off
  wires:
  Switch2/1 -> Pm/1
  I(max)/1 -> Switch1/3, Compare To Constant1/1
  Constant2/1 -> Switch2/1
  Compare To Constant2/1 -> Switch2/2
  Gain/1 -> Switch2/3, Compare To Constant2/1
  Constant3/1 -> Switch3/1
  Compare To Constant3/1 -> Switch3/2
  Switch1/1 -> Im/1
  Compare To Constant1/1 -> Switch1/2
  Constant1/1 -> Switch1/1
  Compare To Constant/1 -> Switch/2
  V(max)/1 -> Switch/3, Compare To Constant/1
  Constant/1 -> Switch/1
  Switch/1 -> Vm/1
  P(max)/1 -> Gain/1
  Rs1/1 -> Switch3/3, Compare To Constant3/1
  Switch3/1 -> Rs/1

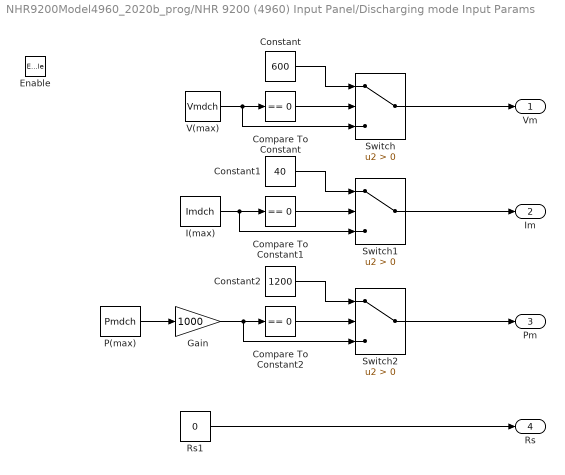
== system NHR9200Model4960_2020b_prog/NHR 9200 (4960) Input Panel/Discharging mode Input Params ==
  Enable : EnablePort
  Compare To Constant : simulink/Logic and Bit Operations/Compare To Constant  relop===  const=0  OutDataTypeStr=boolean
  Compare To Constant1 : simulink/Logic and Bit Operations/Compare To Constant  relop===  const=0  OutDataTypeStr=boolean
  Compare To Constant2 : simulink/Logic and Bit Operations/Compare To Constant  relop===  const=0  OutDataTypeStr=boolean
  Constant : Constant  Value=600
  Constant1 : Constant  Value=40
  Constant2 : Constant  Value=1200
  Gain : Gain  Gain=1000
  I(max) : Constant  Value=Imdch
  P(max) : Constant  Value=Pmdch
  Rs1 : Constant  Value=0
  Switch : Switch  Criteria=u2 > Threshold
  Switch1 : Switch  Criteria=u2 > Threshold
  Switch2 : Switch  Criteria=u2 > Threshold
  V(max) : Constant  Value=Vmdch
  Vm : Outport  VectorParamsAs1DForOutWhenUnconnected=off
  Im : Outport  Port=2  VectorParamsAs1DForOutWhenUnconnected=off
  Pm : Outport  Port=3  VectorParamsAs1DForOutWhenUnconnected=off
  Rs : Outport  Port=4  VectorParamsAs1DForOutWhenUnconnected=off
  wires:
  Rs1/1 -> Rs/1
  P(max)/1 -> Gain/1
  Switch/1 -> Vm/1
  Constant/1 -> Switch/1
  V(max)/1 -> Compare To Constant/1, Switch/3
  Compare To Constant/1 -> Switch/2
  Constant1/1 -> Switch1/1
  Compare To Constant1/1 -> Switch1/2
  Switch1/1 -> Im/1
  Gain/1 -> Compare To Constant2/1, Switch2/3
  Compare To Constant2/1 -> Switch2/2
  Constant2/1 -> Switch2/1
  I(max)/1 -> Compare To Constant1/1, Switch1/3
  Switch2/1 -> Pm/1

== system NHR9200Model4960_2020b_prog/NHR 9200 Safety Settings/Charge safety limits ==
  I : Inport
  P : Inport  Port=2
  Enable : EnablePort
  Trip signal generator (max) Charge Current : Subsystem  mask{trip_thres=Imaxch, trip_t=Timaxch}
      mask prompts: trip_thres "Tripping Threshold (max)"; trip_t "Trip Time"
  Trip signal generator (max) Charge Power : Subsystem  mask{trip_thres=Pmaxch, trip_t=Tpmaxch}
      mask prompts: trip_thres "Tripping Threshold (max)"; trip_t "Trip Time"
  Unit Delay1 : UnitDelay  InitialCondition=1  SampleTime=-1  HasFrameUpgradeWarning=on
  Unit Delay2 : UnitDelay  InitialCondition=1  SampleTime=-1  HasFrameUpgradeWarning=on
  I_trip : Outport  VectorParamsAs1DForOutWhenUnconnected=off
  P_trip : Outport  Port=2  VectorParamsAs1DForOutWhenUnconnected=off
  wires:
  I/1 -> Trip signal generator (max) Charge Current/1(signal_in)
  P/1 -> Trip signal generator (max) Charge Power/1(signal_in)
  Trip signal generator (max) Charge Current/1(signal_trip) -> Unit Delay2/1
  Trip signal generator (max) Charge Power/1(signal_trip) -> Unit Delay1/1
  Unit Delay2/1 -> I_trip/1
  Unit Delay1/1 -> P_trip/1

== system NHR9200Model4960_2020b_prog/NHR 9200 Safety Settings/Discharge safety limits ==
  I : Inport
  P : Inport  Port=2
  Enable : EnablePort
  Trip signal generator (max) Discharge Current : Subsystem  mask{trip_thres=Imaxdch, trip_t=Timaxdch}
      mask prompts: trip_thres "Tripping Threshold (max)"; trip_t "Trip Time"
  Trip signal generator (max) Discharge Power : Subsystem  mask{trip_thres=Pmaxdch, trip_t=Tpmaxdch}
      mask prompts: trip_thres "Tripping Threshold (max)"; trip_t "Trip Time"
  Unit Delay1 : UnitDelay  InitialCondition=1  SampleTime=-1  HasFrameUpgradeWarning=on
  Unit Delay2 : UnitDelay  InitialCondition=1  SampleTime=-1  HasFrameUpgradeWarning=on
  I_trip : Outport  VectorParamsAs1DForOutWhenUnconnected=off
  P_trip : Outport  Port=2  VectorParamsAs1DForOutWhenUnconnected=off
  wires:
  Trip signal generator (max) Discharge Power/1(signal_trip) -> Unit Delay1/1
  I/1 -> Trip signal generator (max) Discharge Current/1(signal_in)
  P/1 -> Trip signal generator (max) Discharge Power/1(signal_in)
  Trip signal generator (max) Discharge Current/1(signal_trip) -> Unit Delay2/1
  Unit Delay2/1 -> I_trip/1
  Unit Delay1/1 -> P_trip/1

== system NHR9200Model4960_2020b_prog/NHR 9200 Safety Settings/Global safety limits ==
  V : Inport
  Trip signal generator (max) Voltage : Subsystem  mask{trip_thres=Vmax, trip_t=Tvmax}
      mask prompts: trip_thres "Tripping Threshold (max)"; trip_t "Trip Time"
  Trip signal generator (min) Voltage : Subsystem  mask{trip_thres=Vmin, trip_t=Tvmin}
      mask prompts: trip_thres "Tripping Threshold (max)"; trip_t "Trip Time"
  Vmin_trip : Outport  VectorParamsAs1DForOutWhenUnconnected=off
  Vmax_trip1 : Outport  Port=2  VectorParamsAs1DForOutWhenUnconnected=off
  wires:
  V/1 -> Trip signal generator (min) Voltage/1(signal_in), Trip signal generator (max) Voltage/1(signal_in)
  Trip signal generator (min) Voltage/1(signal_trip) -> Vmin_trip/1
  Trip signal generator (max) Voltage/1(signal_trip) -> Vmax_trip1/1

== system NHR9200Model4960_2020b_prog/NHR 9200/NHR 9200 Charging mode/source_control ==
  Iout : Inport
  Pout : Inport  Port=2
  Vout : Inport  Port=3
  Pm : Inport  Port=4
  Vm : Inport  Port=5
  Im : Inport  Port=6
  Enable : EnablePort
  Current Slew : RateLimiter  RisingSlewLimit=Islew  FallingSlewLimit=-Islew
  MATLAB Function : MATLAB Function  TreatAsAtomicUnit=on
  Memory : Memory
  Power Slew : RateLimiter  RisingSlewLimit=Pslew  FallingSlewLimit=-Pslew
  Sum : Sum  Inputs=-+
  Sum1 : Sum  Inputs=-+
  Sum2 : Sum  Inputs=-+
  Voltage Slew : RateLimiter  RisingSlewLimit=Vslew  FallingSlewLimit=-Vslew
  Vin : Outport  VectorParamsAs1DForOutWhenUnconnected=off
  wires:
  Vout/1 -> Sum/1
  Iout/1 -> Sum2/1
  Pout/1 -> Sum1/1
  MATLAB Function/1(y) -> Memory/1, Vin/1
  Pm/1 -> Power Slew/1
  Im/1 -> Current Slew/1
  Current Slew/1 -> Sum2/2
  Memory/1 -> MATLAB Function/4(x)
  Sum/1 -> MATLAB Function/2(v)
  Vm/1 -> Voltage Slew/1
  Sum1/1 -> MATLAB Function/1(p)
  Voltage Slew/1 -> Sum/2
  Sum2/1 -> MATLAB Function/3(i)
  Power Slew/1 -> Sum1/2

== system NHR9200Model4960_2020b_prog/NHR 9200/NHR 9200 Discharging mode1/sink_control ==
  Iout : Inport
  Pout : Inport  Port=2
  Pset : Inport  Port=3
  Iset : Inport  Port=4
  Enable : EnablePort
  Current Slew : RateLimiter  RisingSlewLimit=Islew  FallingSlewLimit=-Islew
  Gain2 : Gain  Gain=-1
  MATLAB Function1 : MATLAB Function  TreatAsAtomicUnit=on
  Memory : Memory
  Power Slew : RateLimiter  RisingSlewLimit=Pslew  FallingSlewLimit=-Pslew
  Sum1 : Sum  Inputs=-+
  Sum2 : Sum  Inputs=-+
  Unit Delay2 : UnitDelay  InitialCondition=1  SampleTime=-1  HasFrameUpgradeWarning=on
  Rin : Outport  VectorParamsAs1DForOutWhenUnconnected=off
  wires:
  Power Slew/1 -> Sum1/2
  Sum2/1 -> MATLAB Function1/2(i)
  Sum1/1 -> MATLAB Function1/1(p)
  Memory/1 -> MATLAB Function1/3(x)
  Current Slew/1 -> Sum2/2
  Iset/1 -> Current Slew/1
  Pset/1 -> Power Slew/1
  Iout/1 -> Sum2/1
  Pout/1 -> Sum1/1
  MATLAB Function1/1(y) -> Unit Delay2/1, Memory/1
  Gain2/1 -> Rin/1
  Unit Delay2/1 -> Gain2/1

== system NHR9200Model4960_2020b_prog/NHR 9200 Safety Settings/Charge safety limits/Trip signal generator (max) Charge Current ==
  signal_in : Inport
  trip signal gen : Subsystem
  signal_trip : Outport  VectorParamsAs1DForOutWhenUnconnected=off
  wires:
  trip signal gen/1(trip_out) -> signal_trip/1
  signal_in/1 -> trip signal gen/1(signal in)

== system NHR9200Model4960_2020b_prog/NHR 9200 Safety Settings/Charge safety limits/Trip signal generator (max) Charge Power ==
  signal_in : Inport
  trip signal gen : Subsystem
  signal_trip : Outport  VectorParamsAs1DForOutWhenUnconnected=off
  wires:
  signal_in/1 -> trip signal gen/1(signal in)
  trip signal gen/1(trip_out) -> signal_trip/1

== system NHR9200Model4960_2020b_prog/NHR 9200 Safety Settings/Discharge safety limits/Trip signal generator (max) Discharge Current ==
  signal_in : Inport
  trip signal gen : Subsystem
  signal_trip : Outport  VectorParamsAs1DForOutWhenUnconnected=off
  wires:
  signal_in/1 -> trip signal gen/1(signal in)
  trip signal gen/1(trip_out) -> signal_trip/1

== system NHR9200Model4960_2020b_prog/NHR 9200 Safety Settings/Discharge safety limits/Trip signal generator (max) Discharge Power ==
  signal_in : Inport
  trip signal gen : Subsystem
  signal_trip : Outport  VectorParamsAs1DForOutWhenUnconnected=off
  wires:
  trip signal gen/1(trip_out) -> signal_trip/1
  signal_in/1 -> trip signal gen/1(signal in)

== system NHR9200Model4960_2020b_prog/NHR 9200 Safety Settings/Global safety limits/Trip signal generator (max) Voltage ==
  signal_in : Inport
  trip signal gen : Subsystem
  signal_trip : Outport  VectorParamsAs1DForOutWhenUnconnected=off
  wires:
  signal_in/1 -> trip signal gen/1(signal in)
  trip signal gen/1(trip_out) -> signal_trip/1

== system NHR9200Model4960_2020b_prog/NHR 9200 Safety Settings/Global safety limits/Trip signal generator (min) Voltage ==
  signal_in : Inport
  trip signal gen : Subsystem
  signal_trip : Outport  VectorParamsAs1DForOutWhenUnconnected=off
  wires:
  trip signal gen/1(trip_out) -> signal_trip/1
  signal_in/1 -> trip signal gen/1(signal in)

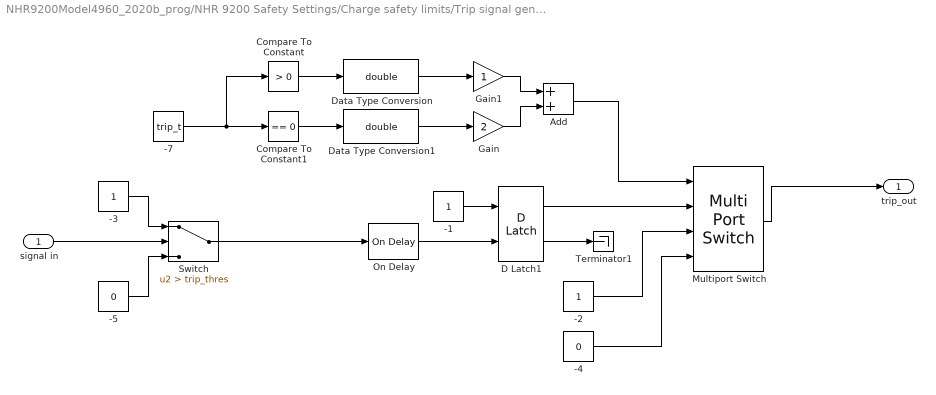
== system NHR9200Model4960_2020b_prog/NHR 9200 Safety Settings/Charge safety limits/Trip signal generator (max) Charge Current/trip signal gen ==
  signal in : Inport
  -1 : Constant  OutDataTypeStr=boolean
  -2 : Constant  OutDataTypeStr=boolean
  -3 : Constant  OutDataTypeStr=boolean
  -4 : Constant  Value=0  OutDataTypeStr=boolean
  -5 : Constant  Value=0  OutDataTypeStr=boolean
  -7 : Constant  Value=trip_t  OutDataTypeStr=boolean
  Add : Sum
  Compare To Constant : simulink/Logic and Bit Operations/Compare To Constant  relop=>  const=0  OutDataTypeStr=uint8
  Compare To Constant1 : simulink/Logic and Bit Operations/Compare To Constant  relop===  const=0  OutDataTypeStr=uint8
  D Latch1 : simulink_extras/Flip Flops/D Latch
      settings: SourceProductBaseCode=SL
  Data Type Conversion : DataTypeConversion  OutDataTypeStr=double
  Data Type Conversion1 : DataTypeConversion  OutDataTypeStr=double
  Gain : Gain  Gain=2
  Gain1 : Gain
  Multiport Switch : MultiPortSwitch  Inputs=2  DataPortForDefault=Additional data port
  On Delay : powerlib_meascontrol/Logic/On Delay  DelayType=On delay  delay=trip_t  ic=0  Ts=0
  Switch : Switch  Criteria=u2 > Threshold  Threshold=trip_thres
  Terminator1 : Terminator
  trip_out : Outport  VectorParamsAs1DForOutWhenUnconnected=off
  wires:
  signal in/1 -> Switch/2
  D Latch1/2 -> Terminator1/1
  -5/1 -> Switch/3
  -3/1 -> Switch/1
  -2/1 -> Multiport Switch/3
  Multiport Switch/1 -> trip_out/1
  -4/1 -> Multiport Switch/4
  D Latch1/1 -> Multiport Switch/2
  On Delay/1 -> D Latch1/2
  Switch/1 -> On Delay/1
  -7/1 -> Compare To Constant1/1, Compare To Constant/1
  Gain1/1 -> Add/1
  Data Type Conversion/1 -> Gain1/1
  Add/1 -> Multiport Switch/1
  Gain/1 -> Add/2
  Data Type Conversion1/1 -> Gain/1
  Compare To Constant1/1 -> Data Type Conversion1/1
  Compare To Constant/1 -> Data Type Conversion/1
  -1/1 -> D Latch1/1

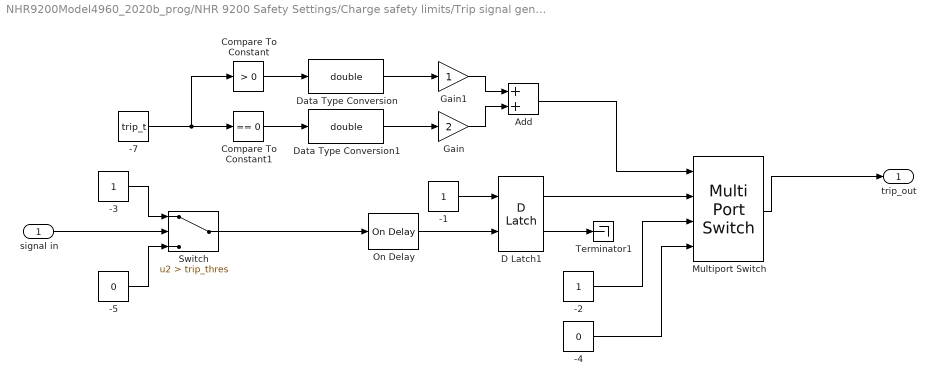
== system NHR9200Model4960_2020b_prog/NHR 9200 Safety Settings/Charge safety limits/Trip signal generator (max) Charge Power/trip signal gen ==
  signal in : Inport
  -1 : Constant  OutDataTypeStr=boolean
  -2 : Constant  OutDataTypeStr=boolean
  -3 : Constant  OutDataTypeStr=boolean
  -4 : Constant  Value=0  OutDataTypeStr=boolean
  -5 : Constant  Value=0  OutDataTypeStr=boolean
  -7 : Constant  Value=trip_t  OutDataTypeStr=boolean
  Add : Sum
  Compare To Constant : simulink/Logic and Bit Operations/Compare To Constant  relop=>  const=0  OutDataTypeStr=uint8
  Compare To Constant1 : simulink/Logic and Bit Operations/Compare To Constant  relop===  const=0  OutDataTypeStr=uint8
  D Latch1 : simulink_extras/Flip Flops/D Latch
      settings: SourceProductBaseCode=SL
  Data Type Conversion : DataTypeConversion  OutDataTypeStr=double
  Data Type Conversion1 : DataTypeConversion  OutDataTypeStr=double
  Gain : Gain  Gain=2
  Gain1 : Gain
  Multiport Switch : MultiPortSwitch  Inputs=2  DataPortForDefault=Additional data port
  On Delay : powerlib_meascontrol/Logic/On Delay  DelayType=On delay  delay=trip_t  ic=0  Ts=0
  Switch : Switch  Criteria=u2 > Threshold  Threshold=trip_thres
  Terminator1 : Terminator
  trip_out : Outport  VectorParamsAs1DForOutWhenUnconnected=off
  wires:
  Switch/1 -> On Delay/1
  On Delay/1 -> D Latch1/2
  D Latch1/1 -> Multiport Switch/2
  -4/1 -> Multiport Switch/4
  Multiport Switch/1 -> trip_out/1
  -2/1 -> Multiport Switch/3
  -3/1 -> Switch/1
  -5/1 -> Switch/3
  D Latch1/2 -> Terminator1/1
  signal in/1 -> Switch/2
  -7/1 -> Compare To Constant1/1, Compare To Constant/1
  Gain1/1 -> Add/1
  Data Type Conversion/1 -> Gain1/1
  Gain/1 -> Add/2
  Data Type Conversion1/1 -> Gain/1
  Compare To Constant1/1 -> Data Type Conversion1/1
  Compare To Constant/1 -> Data Type Conversion/1
  Add/1 -> Multiport Switch/1
  -1/1 -> D Latch1/1

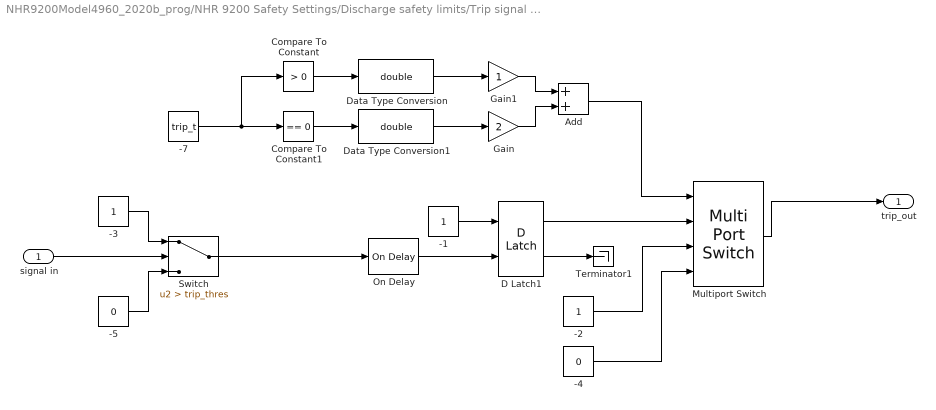
== system NHR9200Model4960_2020b_prog/NHR 9200 Safety Settings/Discharge safety limits/Trip signal generator (max) Discharge Current/trip signal gen ==
  signal in : Inport
  -1 : Constant  OutDataTypeStr=boolean
  -2 : Constant  OutDataTypeStr=boolean
  -3 : Constant  OutDataTypeStr=boolean
  -4 : Constant  Value=0  OutDataTypeStr=boolean
  -5 : Constant  Value=0  OutDataTypeStr=boolean
  -7 : Constant  Value=trip_t  OutDataTypeStr=boolean
  Add : Sum
  Compare To Constant : simulink/Logic and Bit Operations/Compare To Constant  relop=>  const=0  OutDataTypeStr=uint8
  Compare To Constant1 : simulink/Logic and Bit Operations/Compare To Constant  relop===  const=0  OutDataTypeStr=uint8
  D Latch1 : simulink_extras/Flip Flops/D Latch
      settings: SourceProductBaseCode=SL
  Data Type Conversion : DataTypeConversion  OutDataTypeStr=double
  Data Type Conversion1 : DataTypeConversion  OutDataTypeStr=double
  Gain : Gain  Gain=2
  Gain1 : Gain
  Multiport Switch : MultiPortSwitch  Inputs=2  DataPortForDefault=Additional data port
  On Delay : powerlib_meascontrol/Logic/On Delay  DelayType=On delay  delay=trip_t  ic=0  Ts=0
  Switch : Switch  Criteria=u2 > Threshold  Threshold=trip_thres
  Terminator1 : Terminator
  trip_out : Outport  VectorParamsAs1DForOutWhenUnconnected=off
  wires:
  Switch/1 -> On Delay/1
  On Delay/1 -> D Latch1/2
  D Latch1/1 -> Multiport Switch/2
  -4/1 -> Multiport Switch/4
  Multiport Switch/1 -> trip_out/1
  -2/1 -> Multiport Switch/3
  -3/1 -> Switch/1
  -5/1 -> Switch/3
  D Latch1/2 -> Terminator1/1
  signal in/1 -> Switch/2
  -7/1 -> Compare To Constant1/1, Compare To Constant/1
  Gain1/1 -> Add/1
  Data Type Conversion/1 -> Gain1/1
  Gain/1 -> Add/2
  Data Type Conversion1/1 -> Gain/1
  Compare To Constant1/1 -> Data Type Conversion1/1
  Compare To Constant/1 -> Data Type Conversion/1
  Add/1 -> Multiport Switch/1
  -1/1 -> D Latch1/1

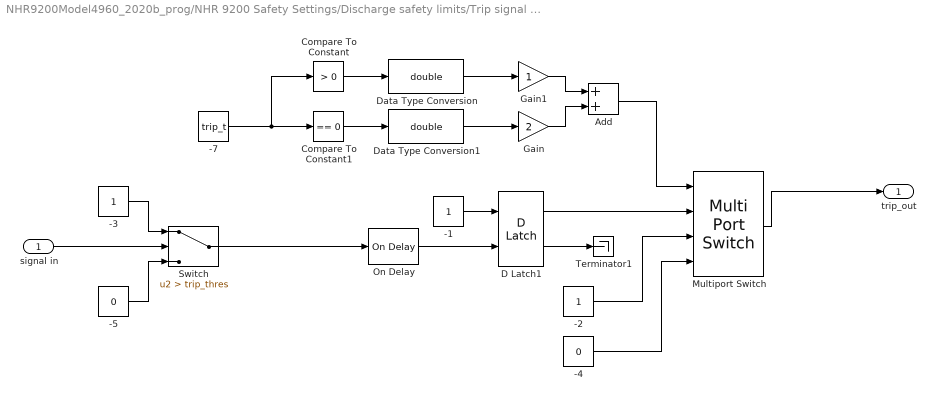
== system NHR9200Model4960_2020b_prog/NHR 9200 Safety Settings/Discharge safety limits/Trip signal generator (max) Discharge Power/trip signal gen ==
  signal in : Inport
  -1 : Constant  OutDataTypeStr=boolean
  -2 : Constant  OutDataTypeStr=boolean
  -3 : Constant  OutDataTypeStr=boolean
  -4 : Constant  Value=0  OutDataTypeStr=boolean
  -5 : Constant  Value=0  OutDataTypeStr=boolean
  -7 : Constant  Value=trip_t  OutDataTypeStr=boolean
  Add : Sum
  Compare To Constant : simulink/Logic and Bit Operations/Compare To Constant  relop=>  const=0  OutDataTypeStr=uint8
  Compare To Constant1 : simulink/Logic and Bit Operations/Compare To Constant  relop===  const=0  OutDataTypeStr=uint8
  D Latch1 : simulink_extras/Flip Flops/D Latch
      settings: SourceProductBaseCode=SL
  Data Type Conversion : DataTypeConversion  OutDataTypeStr=double
  Data Type Conversion1 : DataTypeConversion  OutDataTypeStr=double
  Gain : Gain  Gain=2
  Gain1 : Gain
  Multiport Switch : MultiPortSwitch  Inputs=2  DataPortForDefault=Additional data port
  On Delay : powerlib_meascontrol/Logic/On Delay  DelayType=On delay  delay=trip_t  ic=0  Ts=0
  Switch : Switch  Criteria=u2 > Threshold  Threshold=trip_thres
  Terminator1 : Terminator
  trip_out : Outport  VectorParamsAs1DForOutWhenUnconnected=off
  wires:
  signal in/1 -> Switch/2
  D Latch1/2 -> Terminator1/1
  -5/1 -> Switch/3
  -3/1 -> Switch/1
  -2/1 -> Multiport Switch/3
  Multiport Switch/1 -> trip_out/1
  -4/1 -> Multiport Switch/4
  D Latch1/1 -> Multiport Switch/2
  On Delay/1 -> D Latch1/2
  Switch/1 -> On Delay/1
  -7/1 -> Compare To Constant1/1, Compare To Constant/1
  Gain1/1 -> Add/1
  Data Type Conversion/1 -> Gain1/1
  Gain/1 -> Add/2
  Data Type Conversion1/1 -> Gain/1
  Compare To Constant1/1 -> Data Type Conversion1/1
  Compare To Constant/1 -> Data Type Conversion/1
  Add/1 -> Multiport Switch/1
  -1/1 -> D Latch1/1
